simulink model "optimization_function"  (R2018a)
settings: Solver=VariableStepAuto  StartTime=0.0  StopTime=10.0  RelTol=1e-3
settings Model: Creator=root  LastModifiedBy=root

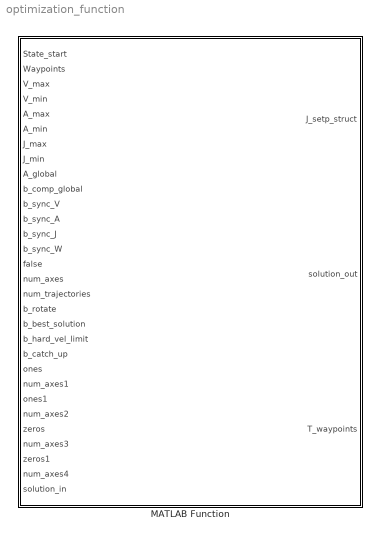
== system optimization_function ==
  MATLAB Function : MATLAB Function  TreatAsAtomicUnit=on

== matlab function optimization_function/MATLAB Function ==
  data: State_start input; J_setp_struct output; Waypoints input; V_max input; V_min input; A_max input; A_min input; J_max input; J_min input; A_global input; b_comp_global input; b_sync_V input; b_sync_A input; b_sync_J input; b_sync_W input; false input; num_axes input; num_trajectories input; b_rotate input; b_best_solution input; b_hard_vel_limit input; b_catch_up input; ones input; num_axes1 input; ones1 input; num_axes2 input; zeros input; num_axes3 input; zeros1 input; num_axes4 input; solution_in input; solution_out output; T_waypoints output
function [J_setp_struct,solution_out,T_waypoints]=  opt_control_mex(State_start,Waypoints,V_max,V_min,A_max,A_min,J_max,J_min,A_global,b_comp_global,b_sync_V,b_sync_A,b_sync_J,b_sync_W,false,num_axes,num_trajectories,b_rotate, b_best_solution,b_hard_vel_limit,b_catch_up,ones,num_axes1,ones1,     num_axes2,zeros,   num_axes3,zeros1,   num_axes4,solution_in)
